simulink model "lineFollowSim_real"  (R2022a)
settings: Solver=FixedStepAuto  StartTime=0.0  StopTime=10.0  RelTol=1e-3  EnableMultiTasking=on
undefined symbols (not defined in the file): InputPWM, WheelSpeed
libraries: arduinolib x8, mobileRoboticsTrainingLib x1
settings Model: ExtModeTrigDuration=2  Creator=heath  LastModifiedBy=heath
settings OptimizationCC: EnhancedBackFolding=on  PassReuseOutputArgsAs=Individual arguments  ZeroExternalMemoryAtStartup=off  ZeroInternalMemoryAtStartup=off  MaxStackSize=64  OptimizeBlockOrder=speed  DifferentSizesBufferReuse=on  OptimizationCustomize=off  EfficientTunableParamExpr=on
settings DebuggingCC: MultiTaskDSMMsg=none  ParameterTunabilityLossMsg=error
settings HardwareCC: ProdBitPerPointer=32  ProdBitPerSizeT=32  ProdBitPerPtrDiffT=32  ProdLargestAtomicInteger=Long  ProdLargestAtomicFloat=Double  ProdWordSize=32  ProdHWDeviceType=ARM Compatible->ARM Cortex  UseEmbeddedCoderFeatures=off  UseSimulinkCoderFeatures=off
settings SFSimCC: MATLABDynamicMemAlloc=off
settings RTWCC: SystemTargetFile=ert.tlc  HardwareBoard=Arduino Nano 33 IoT  TemplateMakefile=ert_default_tmf  Toolchain=Arduino ARM  BuildConfiguration=Faster Runs
settings CodeAppCC: ForceParamTrailComments=on  IgnoreCustomStorageClasses=off  OperatorAnnotations=on  SimulinkDataObjDesc=on  SFDataObjDesc=on  InsertBlockDesc=on
settings ERTTargetCC: SupportContinuousTime=on  SupportNonInlinedSFcns=on  SupportVariableSizeSignals=on  ExtModeTransport=3  ExtModeStaticAlloc=on  ExtModeStaticAllocSize=8192  ExtModeMexFile=ext_xcp  ExtModeIntrfLevel=Level2 - Open

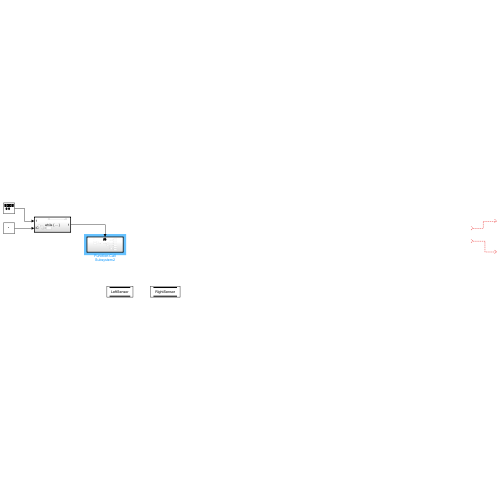
[thumbnail: Simulink's stored preview of the top-level diagram]
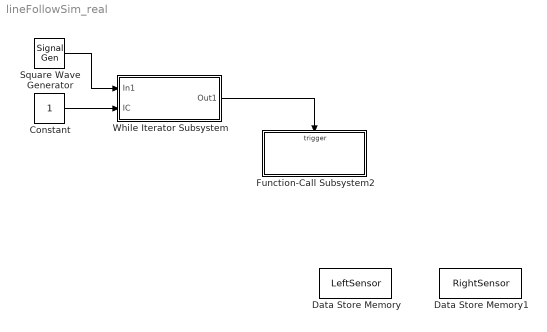
== system lineFollowSim_real ==
  Constant : Constant
  Data Store Memory : DataStoreMemory  DataStoreName=LeftSensor  WriteAfterWriteMsg=warning  ShowAdditionalParam=off
  Data Store Memory1 : DataStoreMemory  DataStoreName=RightSensor  WriteAfterWriteMsg=warning  ShowAdditionalParam=off
  Function-Call Subsystem2 : Subsystem  TreatAsAtomicUnit=on
  Square Wave Generator : SignalGenerator  WaveForm=square  Frequency=100  Units=rad/sec
  While Iterator Subsystem : Subsystem  TreatAsAtomicUnit=on
  wires:
  ? -> ?
  ? -> ?
  While Iterator Subsystem/1(Out1) -> Function-Call Subsystem2/Trigger
  Constant/1 -> While Iterator Subsystem/2(IC)
  Square Wave Generator/1 -> While Iterator Subsystem/1(In1)

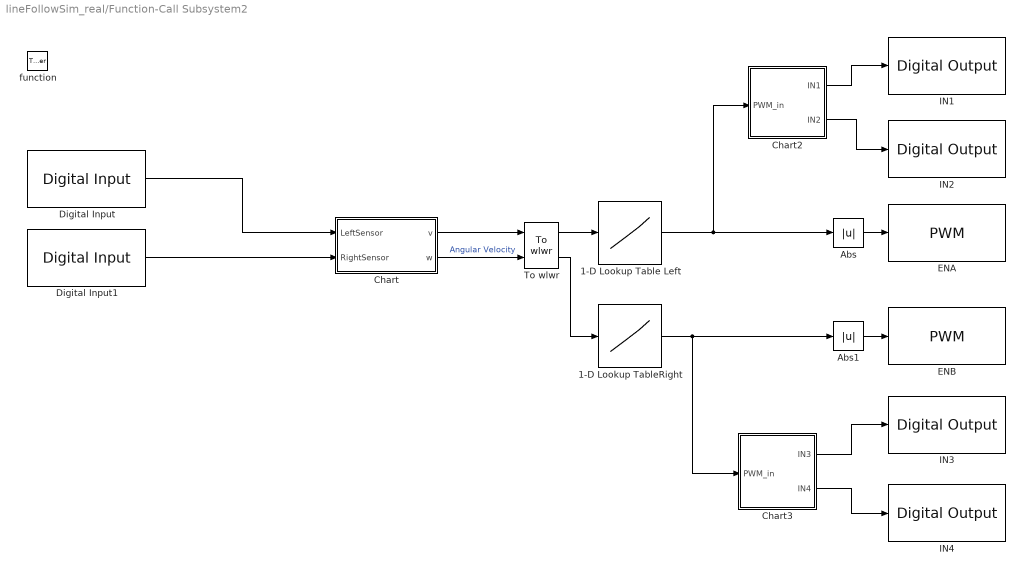
== system lineFollowSim_real/Function-Call Subsystem2 ==
  function : TriggerPort  TriggerType=either  FunctionName=FunctionCallSubsystem2  FunctionVisibility=scoped  VariantControl=(inherit)
  1-D Lookup Table Left : Lookup_n-D  NumberOfTableDimensions=1  BreakpointsForDimension1=WheelSpeed  Table=InputPWM  InternalRulePriority=Speed  RndMeth=Simplest
  1-D Lookup TableRight : Lookup_n-D  NumberOfTableDimensions=1  BreakpointsForDimension1=WheelSpeed  Table=InputPWM  InternalRulePriority=Speed  RndMeth=Simplest
  Abs : Abs  SaturateOnIntegerOverflow=off
  Abs1 : Abs  SaturateOnIntegerOverflow=off
  Chart : Stateflow chart  TreatAsAtomicUnit=on
  Chart2 : Stateflow chart  TreatAsAtomicUnit=on
  Chart3 : Stateflow chart  TreatAsAtomicUnit=on
  Digital Input : arduinolib/Digital Input  pinNumber=12  mode=Default  Direction=input  SampleTime=-1  blockPlatform=arduino
  Digital Input1 : arduinolib/Digital Input  pinNumber=11  mode=Default  Direction=input  SampleTime=-1  blockPlatform=arduino
  ENA : arduinolib/PWM  pinNumber=3  frequencyType=Default  desiredFrequency=490.2  achievableFrequency=490.2
  ENB : arduinolib/PWM  pinNumber=2  frequencyType=Default  desiredFrequency=490.2  achievableFrequency=490.2
  IN1 : arduinolib/Digital Output  pinNumber=4  Direction=output  blockPlatform=arduino
  IN2 : arduinolib/Digital Output  pinNumber=5  Direction=output  blockPlatform=arduino
  IN3 : arduinolib/Digital Output  pinNumber=6  Direction=output  blockPlatform=arduino
  IN4 : arduinolib/Digital Output  pinNumber=7  Direction=output  blockPlatform=arduino
  To wlwr : mobileRoboticsTrainingLib/To wlwr  axleLength=axleLength  wheelR=wheelR
  wires:
  1-D Lookup TableRight/1 -> Chart3/1(PWM_in), Abs1/1
  1-D Lookup Table Left/1 -> Chart2/1(PWM_in), Abs/1
  Abs/1 -> ENA/1
  Chart3/1(IN3) -> IN3/1
  Abs1/1 -> ENB/1
  To wlwr/2 -> 1-D Lookup TableRight/1
  Chart/2(w) -> To wlwr/2  "Angular Velocity"
  Chart/1(v) -> To wlwr/1
  To wlwr/1 -> 1-D Lookup Table Left/1
  Chart3/2(IN4) -> IN4/1
  Digital Input1/1 -> Chart/2(RightSensor)
  Digital Input/1 -> Chart/1(LeftSensor)
  Chart2/1(IN1) -> IN1/1
  Chart2/2(IN2) -> IN2/1

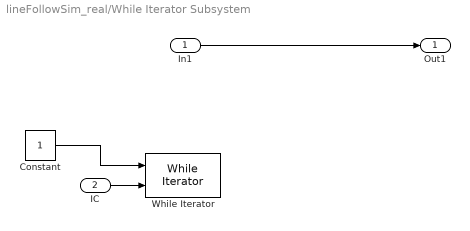
== system lineFollowSim_real/While Iterator Subsystem ==
  In1 : Inport
  IC : Inport  Port=2
  Constant : Constant
  While Iterator : WhileIterator
  Out1 : Outport
  wires:
  IC/1 -> While Iterator/2
  In1/1 -> Out1/1
  Constant/1 -> While Iterator/1

== stateflow chart lineFollowSim_real/Function-Call Subsystem2/Chart3 ==
  state Forward
    entry:
    IN4 = 0;
    IN3 = 1;
  state Back
    entry:
    IN4 = 1;
    IN3 = 0;
  (default) -> Forward
  Forward -> Back : [PWM_in<0]
  Back -> Forward : [PWM_in>=0]
  data: PWM_in input; IN3 output; IN4 output

== stateflow chart lineFollowSim_real/Function-Call Subsystem2/Chart2 ==
  state Forward
    entry:
    IN1 = 1;
    IN2 = 0;
  state Back
    entry:
    IN1 = 0;
    IN2 = 1;
  (default) -> Forward
  Forward -> Back : [PWM_in<0]
  Back -> Forward : [PWM_in>=0]
  data: PWM_in input; IN1 output; IN2 output

== stateflow chart lineFollowSim_real/Function-Call Subsystem2/Chart ==
  (default) -> (junction 47) : % Movement
  (junction 47) -> (junction 48) [order 1] : [LeftSensor>0&&RightSensor>0]
  (junction 47) -> (junction 49) [order 2]
  (junction 48) -> (junction 56) : {v = 0; w = 0;}
  (junction 49) -> (junction 50) [order 1] : [LeftSensor>0]
  (junction 49) -> (junction 51) [order 2]
  (junction 50) -> (junction 55) : {v = 0.1; w = -1;}
  (junction 51) -> (junction 52) [order 1] : [RightSensor>0]
  (junction 51) -> (junction 53) [order 2] : {v = 0.1; w = 0;}
  (junction 52) -> (junction 54) : {v = 0.1; w = 1;}
  (junction 54) -> (junction 53)
  (junction 55) -> (junction 54)
  (junction 56) -> (junction 55)
  (junction 53) -> (junction 57)
  data: LeftSensor input; RightSensor input; v output; w output
